simulink model "pvpanelPaper_4"  (R2020a)
settings: Solver=VariableStepAuto  StartTime=0.0  StopTime=10.0  RelTol=1e-3
libraries: simulink x2
settings Model: Creator=shrad  LastModifiedBy=shrad

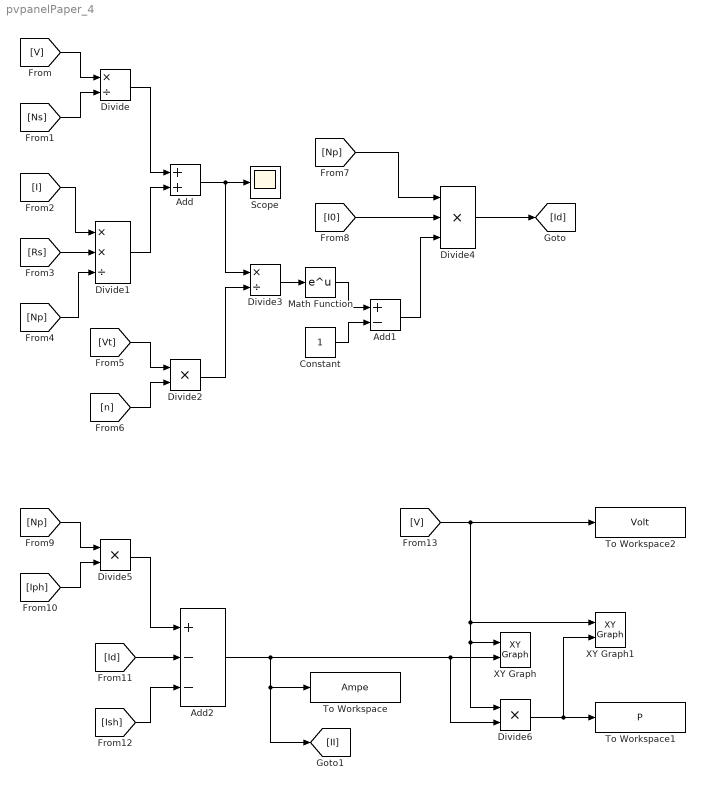
== system pvpanelPaper_4 ==
  Add : Sum
  Add1 : Sum  Inputs=+-
  Add2 : Sum  Inputs=+--
  Constant : Constant
  Divide : Product  Inputs=*/
  Divide1 : Product  Inputs=**/
  Divide2 : Product
  Divide3 : Product  Inputs=*/
  Divide4 : Product  Inputs=3
  Divide5 : Product
  Divide6 : Product
  Math Function : Math  SaturateOnIntegerOverflow=on
  Scope : Scope
  To Workspace : ToWorkspace  VariableName=Ampe  SaveFormat=Timeseries  SampleTime=-1
  To Workspace1 : ToWorkspace  VariableName=P  SaveFormat=Timeseries  SampleTime=-1
  To Workspace2 : ToWorkspace  VariableName=Volt  SaveFormat=Timeseries  SampleTime=-1
  XY Graph : simulink/Sinks/XY Graph  xmin=-1  xmax=1  ymin=-1  ymax=1  st=-1
  XY Graph1 : simulink/Sinks/XY Graph  xmin=-1  xmax=1  ymin=-1  ymax=1  st=-1
  wires:
  [V] -> Divide/1
  [Ns] -> Divide/2
  [Rs] -> Divide1/2
  [Np] -> Divide1/3
  [I] -> Divide1/1
  Divide/1 -> Add/1
  Divide1/1 -> Add/2
  [n] -> Divide2/2
  [Vt] -> Divide2/1
  Add/1 -> Scope/1, Divide3/1
  Divide2/1 -> Divide3/2
  Divide3/1 -> Math Function/1
  Math Function/1 -> Add1/1
  Constant/1 -> Add1/2
  Add1/1 -> Divide4/3
  [I0] -> Divide4/2
  [Np] -> Divide4/1
  Divide4/1 -> [Id]
  [Np] -> Divide5/1
  [Iph] -> Divide5/2
  Divide5/1 -> Add2/1
  [Id] -> Add2/2
  [Ish] -> Add2/3
  Add2/1 -> [II], To Workspace/1, Divide6/2, XY Graph/2
  [V] -> To Workspace2/1, XY Graph1/1, Divide6/1, XY Graph/1
  Divide6/1 -> To Workspace1/1, XY Graph1/2
